simulink model "test_d_v_p_10_1"  (Simulink 7.0)
settings: Solver=ode45  StartTime=0.0  StopTime=30000  RelTol=1e-3
undefined symbols (not defined in the file): BEE2_usr, Down, Up
libraries: xbsIndex_r4 x479, xps_library x33, xbsReplacements_r4 x19, casper_library x15
(part 2 of 4)

== system test_d_v_p_10_1/pulse_ext1 ==
  in : Inport  OutDataType=sfix(16)  OutScaling=2^0
  Constant : xbsIndex_r4/Constant  arith_type=Boolean  const=1  n_bits=1  bin_pt=0  explicit_period=off  period=1  equ=P=C  opselect=C  inp2=PCIN>>17  opr=+  inp1=P  carry=CIN  dbl_ovrd=off  block_type=constant
  Constant17 : xbsIndex_r4/Constant  arith_type=Unsigned  const=pulse_len  n_bits=bits  bin_pt=0  explicit_period=on  period=1  equ=P=C  opselect=C  inp2=PCIN>>17  opr=+  inp1=P  carry=CIN  dbl_ovrd=off  block_type=constant
  Relational1 : xbsIndex_r4/Relational  mode=a<b  en=off  latency=0  dbl_ovrd=off  block_type=relational
      settings: xl_area=[0, 0, 0, 0, 0, 0, 0]  block_version=10.1.3
  Terminator : Terminator
  freeze_cntr : Subsystem  mask{CounterBits=bits}
      mask prompts: CounterBits "Counter Length (2^?)"
  posedge : Subsystem  Tag=Rising Edge Detector
  out : Outport  OutDataType=sfix(16)  OutScaling=2^0
  wires:
  Constant/1 -> freeze_cntr/1(en)
  freeze_cntr/2(we) -> Terminator/1
  freeze_cntr/1(addr) -> Relational1/1
  posedge/1(Out) -> freeze_cntr/2(rst)
  Constant17/1 -> Relational1/2
  Relational1/1 -> out/1
  in/1 -> posedge/1(In)

== system test_d_v_p_10_1/pulse_ext2 ==
  in : Inport  OutDataType=sfix(16)  OutScaling=2^0
  Constant : xbsIndex_r4/Constant  arith_type=Boolean  const=1  n_bits=1  bin_pt=0  explicit_period=off  period=1  equ=P=C  opselect=C  inp2=PCIN>>17  opr=+  inp1=P  carry=CIN  dbl_ovrd=off  block_type=constant
  Constant17 : xbsIndex_r4/Constant  arith_type=Unsigned  const=pulse_len  n_bits=bits  bin_pt=0  explicit_period=on  period=1  equ=P=C  opselect=C  inp2=PCIN>>17  opr=+  inp1=P  carry=CIN  dbl_ovrd=off  block_type=constant
  Relational1 : xbsIndex_r4/Relational  mode=a<b  en=off  latency=0  dbl_ovrd=off  block_type=relational
      settings: xl_area=[0, 0, 0, 0, 0, 0, 0]  block_version=10.1.3
  Terminator : Terminator
  freeze_cntr : Subsystem  mask{CounterBits=bits}
      mask prompts: CounterBits "Counter Length (2^?)"
  posedge : Subsystem  Tag=Rising Edge Detector
  out : Outport  OutDataType=sfix(16)  OutScaling=2^0
  wires:
  Constant/1 -> freeze_cntr/1(en)
  freeze_cntr/2(we) -> Terminator/1
  freeze_cntr/1(addr) -> Relational1/1
  posedge/1(Out) -> freeze_cntr/2(rst)
  Constant17/1 -> Relational1/2
  Relational1/1 -> out/1
  in/1 -> posedge/1(In)

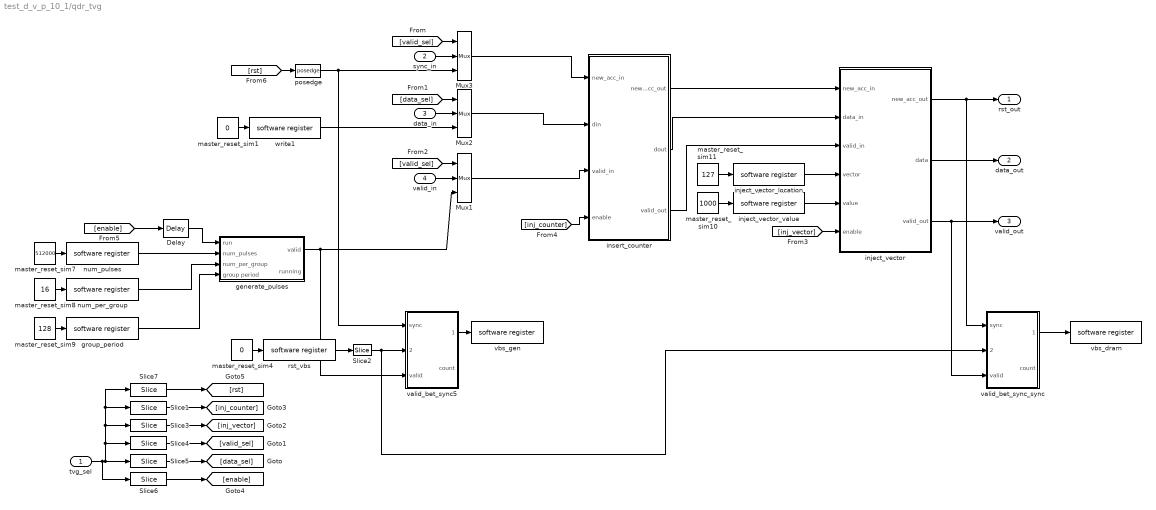
== system test_d_v_p_10_1/qdr_tvg ==
  tvg_sel : Inport  OutDataType=sfix(16)  OutScaling=2^0
  sync_in : Inport  Port=2  OutDataType=sfix(16)  OutScaling=2^0
  data_in : Inport  Port=3  OutDataType=sfix(16)  OutScaling=2^0
  valid_in : Inport  Port=4  OutDataType=sfix(16)  OutScaling=2^0
  Delay : xbsIndex_r4/Delay  en=off  latency=1  dbl_ovrd=off  reg_retiming=on  block_type=delay
      settings: xl_area=[0, 0, 0, 0, 0, 0, 0]
  Mux1 : xbsIndex_r4/Mux  inputs=2  en=off  latency=0  precision=Full  arith_type="Signed  (2's comp)"  n_bits=8  bin_pt=2  quantization=Truncate  overflow=Wrap  dbl_ovrd=off  block_type=mux
      settings: xl_area=[0, 0, 0, 0, 0, 0, 0]
  Mux2 : xbsIndex_r4/Mux  inputs=2  en=off  latency=0  precision=Full  arith_type="Signed  (2's comp)"  n_bits=8  bin_pt=2  quantization=Truncate  overflow=Wrap  dbl_ovrd=off  block_type=mux
      settings: xl_area=[0, 0, 0, 0, 0, 0, 0]
  Mux3 : xbsIndex_r4/Mux  inputs=2  en=off  latency=0  precision=Full  arith_type="Signed  (2's comp)"  n_bits=8  bin_pt=2  quantization=Truncate  overflow=Wrap  dbl_ovrd=off  block_type=mux
      settings: xl_area=[0, 0, 0, 0, 0, 0, 0]
  Slice1 : xbsIndex_r4/Slice  nbits=1  boolean_output=on  mode=Lower Bit Location + Width  bit1=0  base1=MSB of Input  bit0=4  base0=LSB of Input  dbl_ovrd=off  block_type=slice
      settings: infoedit="Extracts a given range of bits from each input sample and presents it at the output.  The output type is ordinarily unsigned with binary point at zero, but can be Boolean when the slice is one bit wide.<P><P>Hardware notes: In hardware this block costs nothing."  block_version=10.1.3
  Slice2 : xbsIndex_r4/Slice  nbits=1  boolean_output=on  mode=Lower Bit Location + Width  bit1=0  base1=MSB of Input  bit0=0  base0=LSB of Input  dbl_ovrd=off  block_type=slice
      settings: infoedit="Extracts a given range of bits from each input sample and presents it at the output.  The output type is ordinarily unsigned with binary point at zero, but can be Boolean when the slice is one bit wide.<P><P>Hardware notes: In hardware this block costs nothing."  block_version=10.1.3
  Slice3 : xbsIndex_r4/Slice  nbits=1  boolean_output=on  mode=Lower Bit Location + Width  bit1=0  base1=MSB of Input  bit0=3  base0=LSB of Input  dbl_ovrd=off  block_type=slice
      settings: infoedit="Extracts a given range of bits from each input sample and presents it at the output.  The output type is ordinarily unsigned with binary point at zero, but can be Boolean when the slice is one bit wide.<P><P>Hardware notes: In hardware this block costs nothing."  block_version=10.1.3
  Slice4 : xbsIndex_r4/Slice  nbits=1  boolean_output=on  mode=Lower Bit Location + Width  bit1=0  base1=MSB of Input  bit0=2  base0=LSB of Input  dbl_ovrd=off  block_type=slice
      settings: infoedit="Extracts a given range of bits from each input sample and presents it at the output.  The output type is ordinarily unsigned with binary point at zero, but can be Boolean when the slice is one bit wide.<P><P>Hardware notes: In hardware this block costs nothing."  block_version=10.1.3
  Slice5 : xbsIndex_r4/Slice  nbits=1  boolean_output=on  mode=Lower Bit Location + Width  bit1=0  base1=MSB of Input  bit0=1  base0=LSB of Input  dbl_ovrd=off  block_type=slice
      settings: infoedit="Extracts a given range of bits from each input sample and presents it at the output.  The output type is ordinarily unsigned with binary point at zero, but can be Boolean when the slice is one bit wide.<P><P>Hardware notes: In hardware this block costs nothing."  block_version=10.1.3
  Slice6 : xbsIndex_r4/Slice  nbits=1  boolean_output=on  mode=Lower Bit Location + Width  bit1=0  base1=MSB of Input  bit0=0  base0=LSB of Input  dbl_ovrd=off  block_type=slice
      settings: infoedit="Extracts a given range of bits from each input sample and presents it at the output.  The output type is ordinarily unsigned with binary point at zero, but can be Boolean when the slice is one bit wide.<P><P>Hardware notes: In hardware this block costs nothing."  block_version=10.1.3
  Slice7 : xbsIndex_r4/Slice  nbits=1  boolean_output=on  mode=Lower Bit Location + Width  bit1=0  base1=MSB of Input  bit0=5  base0=LSB of Input  dbl_ovrd=off  block_type=slice
      settings: infoedit="Extracts a given range of bits from each input sample and presents it at the output.  The output type is ordinarily unsigned with binary point at zero, but can be Boolean when the slice is one bit wide.<P><P>Hardware notes: In hardware this block costs nothing."  block_version=10.1.3
  generate_pulses : Subsystem
  group_period : xps_library/software register  Tag=xps:sw_reg  SystemSampleTime=-1  io_dir=From Processor  arith_type=Unsigned  bitwidth=32  bin_pt=0  sample_period=1  gw_name=test_d_v_p_10_1_qdr_tvg_group_period_user_data_out
      link override qdr_vacc_dram_tvg1_group_period_user_data_out: arith_type=Unsigned  n_bits=32  bin_pt=0  period=1
      link override qdr_vacc_qdr_tvg_group_period_user_data_out: arith_type=Unsigned  n_bits=32  bin_pt=0  period=1
      link override test_qdr_vacc_qdr_tvg_group_period_user_data_out: arith_type=Unsigned  n_bits=32  bin_pt=0  period=1
  inject_vector : Subsystem  mask{num_vectors=len}
      mask prompts: num_vectors "number of vectors"
      mask init:
      | fmtstr = sprintf('Vector Length: %d', num_vectors);
      | set_param(gcb, 'AttributesFormatString', fmtstr);
      settings: AttributesFormatString=Vector Length: 150
  inject_vector_location : xps_library/software register  Tag=xps:sw_reg  SystemSampleTime=-1  io_dir=From Processor  arith_type=Unsigned  bitwidth=32  bin_pt=0  sample_period=1  gw_name=test_d_v_p_10_1_qdr_tvg_inject_vector_location_user_data_out
      link override qdr_vacc_dram_tvg1_inject_vector_location_user_data_out: arith_type=Unsigned  n_bits=32  bin_pt=0  period=1
      link override qdr_vacc_qdr_tvg_inject_vector_location_user_data_out: arith_type=Unsigned  n_bits=32  bin_pt=0  period=1
      link override test_qdr_vacc_qdr_tvg_inject_vector_location_user_data_out: arith_type=Unsigned  n_bits=32  bin_pt=0  period=1
  inject_vector_value : xps_library/software register  Tag=xps:sw_reg  SystemSampleTime=-1  io_dir=From Processor  arith_type="Signed  (2's comp)"  bitwidth=32  bin_pt=0  sample_period=1  gw_name=test_d_v_p_10_1_qdr_tvg_inject_vector_value_user_data_out
      link override qdr_vacc_dram_tvg1_inject_vector_value_user_data_out: arith_type=Unsigned  n_bits=32  bin_pt=0  period=1
      link override qdr_vacc_qdr_tvg_inject_vector_value_user_data_out: arith_type=Unsigned  n_bits=32  bin_pt=0  period=1
      link override test_qdr_vacc_qdr_tvg_inject_vector_value_user_data_out: arith_type="Signed  (2's comp)"  n_bits=32  bin_pt=0  period=1
  insert_counter : Subsystem  mask{vec_len=len}
      mask prompts: vec_len "Vector Length?"
      mask init:
      | fmtstr = sprintf('Vector Length: %d', vec_len);
      | set_param(gcb, 'AttributesFormatString', fmtstr);
      settings: AttributesFormatString=Vector Length: 150
  master_reset_sim1 : Constant  Value=0  OutDataType=sfix(16)  OutScaling=2^0
  master_reset_sim10 : Constant  Value=1000  OutDataType=sfix(16)  OutScaling=2^0
  master_reset_sim11 : Constant  Value=127  OutDataType=sfix(16)  OutScaling=2^0
  master_reset_sim4 : Constant  Value=0  OutDataType=sfix(16)  OutScaling=2^0
  master_reset_sim7 : Constant  Value=512000  OutDataType=sfix(16)  OutScaling=2^0
  master_reset_sim8 : Constant  Value=16  OutDataType=sfix(16)  OutScaling=2^0
  master_reset_sim9 : Constant  Value=128  OutDataType=sfix(16)  OutScaling=2^0
  num_per_group : xps_library/software register  Tag=xps:sw_reg  SystemSampleTime=-1  io_dir=From Processor  arith_type=Unsigned  bitwidth=32  bin_pt=0  sample_period=1  gw_name=test_d_v_p_10_1_qdr_tvg_num_per_group_user_data_out
      link override qdr_vacc_dram_tvg1_num_per_group_user_data_out: arith_type=Unsigned  n_bits=32  bin_pt=0  period=1
      link override qdr_vacc_qdr_tvg_num_per_group_user_data_out: arith_type=Unsigned  n_bits=32  bin_pt=0  period=1
      link override test_qdr_vacc_qdr_tvg_num_per_group_user_data_out: arith_type=Unsigned  n_bits=32  bin_pt=0  period=1
  num_pulses : xps_library/software register  Tag=xps:sw_reg  SystemSampleTime=-1  io_dir=From Processor  arith_type=Unsigned  bitwidth=32  bin_pt=0  sample_period=1  gw_name=test_d_v_p_10_1_qdr_tvg_num_pulses_user_data_out
      link override qdr_vacc_dram_tvg1_num_pulses_user_data_out: arith_type=Unsigned  n_bits=32  bin_pt=0  period=1
      link override qdr_vacc_qdr_tvg_num_pulses_user_data_out: arith_type=Unsigned  n_bits=32  bin_pt=0  period=1
      link override test_qdr_vacc_qdr_tvg_num_pulses_user_data_out: arith_type=Unsigned  n_bits=32  bin_pt=0  period=1
  posedge : casper_library/Misc/posedge  Tag=Rising Edge Detector  SystemSampleTime=-1
  rst_vbs : xps_library/software register  Tag=xps:sw_reg  SystemSampleTime=-1  io_dir=From Processor  arith_type=Unsigned  bitwidth=32  bin_pt=0  sample_period=1  gw_name=test_d_v_p_10_1_qdr_tvg_rst_vbs_user_data_out
      link override qdr_vacc_dram_tvg1_rst_vbs_user_data_out: arith_type=Unsigned  n_bits=32  bin_pt=0  period=1
      link override qdr_vacc_qdr_tvg_rst_vbs_user_data_out: arith_type=Unsigned  n_bits=32  bin_pt=0  period=1
      link override test_qdr_vacc_qdr_tvg_rst_vbs_user_data_out: arith_type=Unsigned  n_bits=32  bin_pt=0  period=1
  valid_bet_sync5 : Subsystem
  valid_bet_sync_sync : Subsystem
  vbs_dram : xps_library/software register  Tag=xps:sw_reg  SystemSampleTime=-1  io_dir=To Processor  arith_type=Unsigned  bitwidth=32  bin_pt=0  sample_period=1  gw_name=test_d_v_p_10_1_qdr_tvg_vbs_dram_user_data_in
      link override convert: arith_type=Unsigned  n_bits=32  bin_pt=0
  vbs_gen : xps_library/software register  Tag=xps:sw_reg  SystemSampleTime=-1  io_dir=To Processor  arith_type=Unsigned  bitwidth=32  bin_pt=0  sample_period=1  gw_name=test_d_v_p_10_1_qdr_tvg_vbs_gen_user_data_in
      link override convert: arith_type=Unsigned  n_bits=32  bin_pt=0
  write1 : xps_library/software register  Tag=xps:sw_reg  SystemSampleTime=-1  io_dir=From Processor  arith_type="Signed  (2's comp)"  bitwidth=32  bin_pt=0  sample_period=1  gw_name=test_d_v_p_10_1_qdr_tvg_write1_user_data_out
      link override qdr_vacc_dram_tvg1_write1_user_data_out: arith_type=Unsigned  n_bits=32  bin_pt=0  period=1
      link override qdr_vacc_qdr_tvg_write1_user_data_out: arith_type=Unsigned  n_bits=32  bin_pt=0  period=1
      link override test_qdr_vacc_qdr_tvg_write1_user_data_out: arith_type="Signed  (2's comp)"  n_bits=32  bin_pt=0  period=1
  rst_out : Outport  OutDataType=sfix(16)  OutScaling=2^0
  data_out : Outport  Port=2  OutDataType=sfix(16)  OutScaling=2^0
  valid_out : Outport  Port=3  OutDataType=sfix(16)  OutScaling=2^0
  wires:
  write1/1 -> Mux2/3
  master_reset_sim1/1 -> write1/1
  [rst] -> posedge/1
  num_pulses/1 -> generate_pulses/2(num_pulses)
  master_reset_sim7/1 -> num_pulses/1
  num_per_group/1 -> generate_pulses/3(num_per_group)
  master_reset_sim8/1 -> num_per_group/1
  group_period/1 -> generate_pulses/4(group period)
  master_reset_sim9/1 -> group_period/1
  Mux1/1 -> insert_counter/3(valid_in)
  valid_in/1 -> Mux1/2
  inject_vector/1(new_acc_out) -> rst_out/1, valid_bet_sync_sync/1(sync)
  inject_vector/2(data) -> data_out/1
  inject_vector/3(valid_out) -> valid_out/1, valid_bet_sync_sync/3(valid)
  insert_counter/1(new_acc_out) -> inject_vector/1(new_acc_in)
  Mux2/1 -> insert_counter/2(din)
  data_in/1 -> Mux2/2
  sync_in/1 -> Mux3/2
  Mux3/1 -> insert_counter/1(new_acc_in)
  Slice5/1 -> [data_sel]
  tvg_sel/1 -> Slice5/1, Slice3/1, Slice1/1, Slice7/1, Slice4/1, Slice6/1
  Slice4/1 -> [valid_sel]
  [valid_sel] -> Mux3/1
  [data_sel] -> Mux2/1
  [valid_sel] -> Mux1/1
  Slice3/1 -> [inj_vector]
  Slice1/1 -> [inj_counter]
  [enable] -> Delay/1
  insert_counter/2(dout) -> inject_vector/2(data_in)
  insert_counter/3(valid_out) -> inject_vector/3(valid_in)
  generate_pulses/1(valid) -> valid_bet_sync5/3(valid), Mux1/3
  posedge/1 -> valid_bet_sync5/1(sync), Mux3/3
  [inj_vector] -> inject_vector/6(enable)
  master_reset_sim11/1 -> inject_vector_location/1
  inject_vector_location/1 -> inject_vector/4(vector)
  master_reset_sim10/1 -> inject_vector_value/1
  inject_vector_value/1 -> inject_vector/5(value)
  [inj_counter] -> insert_counter/4(enable)
  Slice6/1 -> [enable]
  Slice7/1 -> [rst]
  valid_bet_sync5/1(max_count) -> vbs_gen/1
  master_reset_sim4/1 -> rst_vbs/1
  Slice2/1 -> valid_bet_sync5/2(rst_max), valid_bet_sync_sync/2(rst_max)
  rst_vbs/1 -> Slice2/1
  valid_bet_sync_sync/1(max_count) -> vbs_dram/1
  Delay/1 -> generate_pulses/1(run)

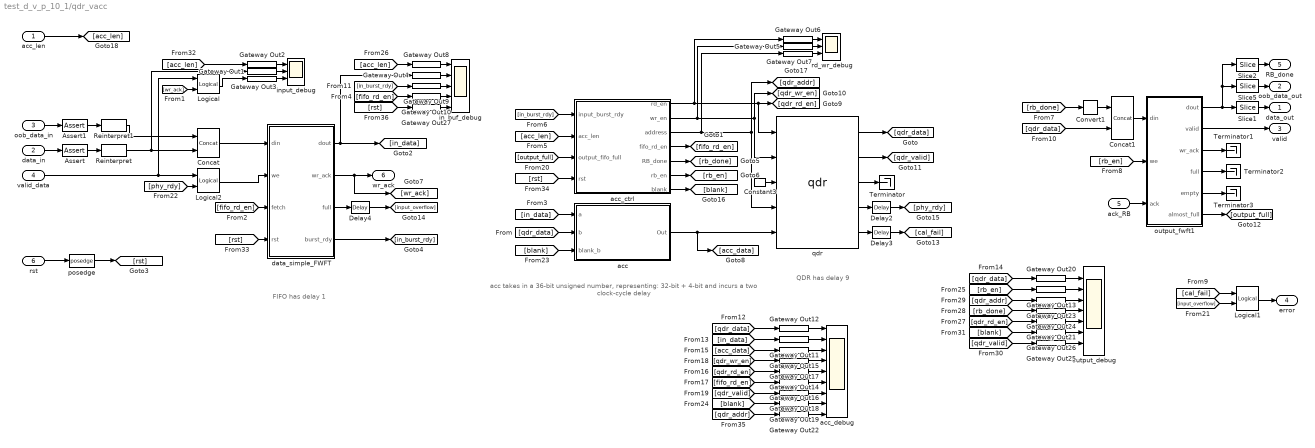
== system test_d_v_p_10_1/qdr_vacc ==
  note: QDR has delay 9
  note: FIFO has delay 1
  note: acc takes in a 36-bit unsigned
      | number, representing:
      | 32-bit + 4-bit and
      | incurs a two clock-cycle delay
  acc_len : Inport  OutDataType=sfix(16)  OutScaling=2^0
  data_in : Inport  Port=2  OutDataType=sfix(16)  OutScaling=2^0
  oob_data_in : Inport  Port=3  OutDataType=sfix(16)  OutScaling=2^0
  valid_data : Inport  Port=4  OutDataType=sfix(16)  OutScaling=2^0
  ack_RB : Inport  Port=5  OutDataType=sfix(16)  OutScaling=2^0
  rst : Inport  Port=6  OutDataType=sfix(16)  OutScaling=2^0
  Assert : xbsIndex_r4/Assert  assert_type=on  type_source=Explicitly  arith_type="Signed  (2's comp)"  n_bits=32  bin_pt=0  assert_rate=off  rate_source=Explicitly  period=1  output_port=on  block_type=assert
      settings: infoedit=Asserts a user-defined sample rate and/or type on a signal.<P><P>Hardware notes: In hardware this block costs nothing.  block_version=10.1.3
  Assert1 : xbsIndex_r4/Assert  assert_type=on  type_source=Explicitly  arith_type=Unsigned  n_bits=4  bin_pt=0  assert_rate=on  rate_source=Explicitly  period=1  output_port=on  block_type=assert
      settings: infoedit=Asserts a user-defined sample rate and/or type on a signal.<P><P>Hardware notes: In hardware this block costs nothing.  block_version=10.1.3
  Concat : xbsIndex_r4/Concat  num_inputs=2  dbl_ovrd=off  block_type=concat
      settings: block_version=9.2.01
  Concat1 : xbsIndex_r4/Concat  num_inputs=2  dbl_ovrd=off  block_type=concat
      settings: block_version=9.2.01
  Constant3 : xbsIndex_r4/Constant  arith_type=Unsigned  const=(2^4)-1  n_bits=4  bin_pt=0  explicit_period=on  period=1  equ=P=C  opselect=C  inp2=PCIN>>17  opr=+  inp1=P  carry=CIN  dbl_ovrd=off  block_type=constant
      settings: block_version=9.2.01
  Convert1 : xbsIndex_r4/Convert  arith_type=Unsigned  n_bits=1  bin_pt=0  quantization=Truncate  overflow=Wrap  latency=0  dbl_ovrd=off  pipeline=off  block_type=convert
      settings: xl_area=[0, 0, 0, 0, 0, 0, 0]  block_version=9.2.01
  Delay2 : xbsIndex_r4/Delay  en=off  latency=2  dbl_ovrd=off  reg_retiming=on  block_type=delay
  Delay3 : xbsIndex_r4/Delay  en=off  latency=2  dbl_ovrd=off  reg_retiming=on  block_type=delay
  Delay4 : xbsIndex_r4/Delay  en=off  latency=2  dbl_ovrd=off  reg_retiming=on  block_type=delay
  Gateway Out{1..27} (27 alike) : xbsIndex_r4/Gateway Out  hdl_port=on  timing_constraint=None  locs_specified=off  LOCs={}  block_type=gatewayout
      settings: infoedit="Gateway out block.  Converts Xilinx fixed point inputs into ouputs of type Simulink integer, double, or fixed point.<P><P>Hardware notes:  In hardware these blocks become top level output ports or are discarded, depending on how they are configured."  xl_area=[0, 0, 0, 0, 0, 0, 0]  block_version=10.1.3
  Logical : xbsIndex_r4/Logical  logical_function=AND  inputs=2  en=off  latency=0  precision=Full  arith_type=Unsigned  n_bits=16  bin_pt=0  align_bp=on  dbl_ovrd=off  block_type=logical
  Logical1 : xbsIndex_r4/Logical  logical_function=OR  inputs=2  en=off  latency=1  precision=Full  arith_type=Unsigned  n_bits=16  bin_pt=0  align_bp=on  dbl_ovrd=off  block_type=logical
  Logical2 : xbsIndex_r4/Logical  logical_function=AND  inputs=2  en=off  latency=0  precision=Full  arith_type=Unsigned  n_bits=16  bin_pt=0  align_bp=on  dbl_ovrd=off  block_type=logical
  Reinterpret : xbsIndex_r4/Reinterpret  force_arith_type=on  arith_type=Unsigned  force_bin_pt=on  bin_pt=0  block_type=reinterpret
      settings: infoedit="Changes signal type without altering the binary representation.   You can changed the signal between signed and unsigned, and relocate the binary point.<P><P>Hardware notes: In hardware this block costs nothing.<P><P>Example:  Suppose the input is 6 bits wide, signed, with 2 fractional bits, and the output is forced to unsigned with 0 fractional bits.  Then an input of -2.0 (1110.00 in binary 2's complement) becomes an output of 56 (111000 in binary)."  block_version=9.2.01
  Reinterpret1 : xbsIndex_r4/Reinterpret  force_arith_type=on  arith_type=Unsigned  force_bin_pt=on  bin_pt=0  block_type=reinterpret
      settings: infoedit="Changes signal type without altering the binary representation.   You can changed the signal between signed and unsigned, and relocate the binary point.<P><P>Hardware notes: In hardware this block costs nothing.<P><P>Example:  Suppose the input is 6 bits wide, signed, with 2 fractional bits, and the output is forced to unsigned with 0 fractional bits.  Then an input of -2.0 (1110.00 in binary 2's complement) becomes an output of 56 (111000 in binary)."  block_version=9.2.01
  Slice1 : xbsIndex_r4/Slice  nbits=32  boolean_output=off  mode=Lower Bit Location + Width  bit1=96  base1=MSB of Input  bit0=0  base0=LSB of Input  dbl_ovrd=off  block_type=slice
      settings: infoedit="Extracts a given range of bits from each input sample and presents it at the output.  The output type is ordinarily unsigned with binary point at zero, but can be Boolean when the slice is one bit wide.<P><P>Hardware notes: In hardware this block costs nothing."  block_version=9.2.01
  Slice2 : xbsIndex_r4/Slice  nbits=1  boolean_output=on  mode=Lower Bit Location + Width  bit1=-1  base1=MSB of Input  bit0=36  base0=LSB of Input  dbl_ovrd=off  block_type=slice
      settings: infoedit="Extracts a given range of bits from each input sample and presents it at the output.  The output type is ordinarily unsigned with binary point at zero, but can be Boolean when the slice is one bit wide.<P><P>Hardware notes: In hardware this block costs nothing."  block_version=9.2.01
  Slice5 : xbsIndex_r4/Slice  nbits=4  boolean_output=off  mode=Lower Bit Location + Width  bit1=96  base1=MSB of Input  bit0=32  base0=LSB of Input  dbl_ovrd=off  block_type=slice
      settings: infoedit="Extracts a given range of bits from each input sample and presents it at the output.  The output type is ordinarily unsigned with binary point at zero, but can be Boolean when the slice is one bit wide.<P><P>Hardware notes: In hardware this block costs nothing."  block_version=9.2.01
  Terminator{,1..3} (4 alike) : Terminator
  acc : Subsystem
  acc_ctrl : Subsystem
  acc_debug : Scope  NumInputPorts=9
      settings: TimeRange=57000  YMin=0~0~0~0~0~0~0~0~0  YMax=3000~1000~3000~1~1~1~1~1~150  SaveName=ScopeData4
  data_simple_FWFT : Subsystem  mask{burst_bits=burst_bits}
      mask prompts: burst_bits "Burst Length (2^?)"
      mask help: A rollback fifo behaves as a normal fifo, except that data which are written in have to be "committed" before they become available for readout. Moreover, any data which are written in and have not been committed can be "discarded", and will never be made available for readout.
      mask init:
      | fmtstr = sprintf('Depth: %d', 2^(burst_bits+2));
      | set_param(gcb, 'AttributesFormatString', fmtstr);
      settings: AttributesFormatString=Depth: 64
  in_buf_debug : Scope  NumInputPorts=5
      settings: YMin=12000~0~-5~-5~-5  YMax=13300~1~5~5~5  SaveName=ScopeData2
  input_debug : Scope  NumInputPorts=3
      settings: YMin=12000~0~-5  YMax=13300~1~5
  output_debug : Scope  NumInputPorts=7
      settings: YMin=0~0~0~0~0~0~0  YMax=600~1~225~1~1~1~1  SaveName=ScopeData3
  output_fwft1 : Subsystem  mask{depth_bits=10, burst_bits=burst_bits}
      mask prompts: depth_bits "Fifo Depth (2^?):"; burst_bits "Almost full warning (2^?)"
      mask help: A rollback fifo behaves as a normal fifo, except that data which are written in have to be "committed" before they become available for readout. Moreover, any data which are written in and have not been committed can be "discarded", and will never be made available for readout.
      mask init:
      | fmtstr = sprintf('Depth: %d', 2^depth_bits);
      | set_param(gcb, 'AttributesFormatString', fmtstr);
      settings: AttributesFormatString=Depth: 1024
  posedge : casper_library/Misc/posedge  Tag=Rising Edge Detector  SystemSampleTime=-1
  qdr : xps_library/qdr  Tag=xps:qdr  SystemSampleTime=-1  which_qdr=qdr0  qdr_awidth=12
  rd_wr_debug : Scope  NumInputPorts=3
      settings: YMin=12000~0~-5  YMax=13300~1~5
  data_out : Outport  OutDataType=sfix(16)  OutScaling=2^0
  oob_data_out : Outport  Port=2  OutDataType=sfix(16)  OutScaling=2^0
  valid : Outport  Port=3  OutDataType=sfix(16)  OutScaling=2^0
  error : Outport  Port=4  OutDataType=sfix(16)  OutScaling=2^0
  RB_done : Outport  Port=5  OutDataType=sfix(16)  OutScaling=2^0
  wr_ack : Outport  Port=6  OutDataType=sfix(16)  OutScaling=2^0
  wires:
  data_in/1 -> Assert/1
  valid_data/1 -> Logical/1, Logical2/1
  Concat/1 -> data_simple_FWFT/1(din)
  data_simple_FWFT/2(wr_ack) -> wr_ack/1, [wr_ack]
  acc_ctrl/1(rd_en) -> Gateway Out6/1, [qdr_rd_en], qdr/1
  acc_ctrl/2(wr_en) -> Gateway Out5/1, [qdr_wr_en], qdr/2
  acc_ctrl/3(address) -> Gateway Out7/1, [qdr_addr], qdr/4
  qdr/1 -> [qdr_data]
  Constant3/1 -> qdr/3
  acc_ctrl/4(fifo_rd_en) -> [fifo_rd_en]
  [fifo_rd_en] -> data_simple_FWFT/3(fetch)
  data_simple_FWFT/1(dout) -> Gateway Out4/1, [in_data]
  [in_burst_rdy] -> acc_ctrl/1(input_burst_rdy)
  data_simple_FWFT/4(burst_rdy) -> [in_burst_rdy]
  output_fwft1/2(valid) -> valid/1
  ack_RB/1 -> output_fwft1/3(ack)
  [rb_en] -> output_fwft1/2(we)
  [qdr_data] -> Concat1/2
  Concat1/1 -> output_fwft1/1(din)
  [rb_done] -> Convert1/1
  Convert1/1 -> Concat1/1
  output_fwft1/1(dout) -> Slice1/1, Slice2/1, Slice5/1
  Slice2/1 -> RB_done/1
  Slice1/1 -> data_out/1
  Gateway Out6/1 -> rd_wr_debug/1
  Gateway Out5/1 -> rd_wr_debug/2
  Gateway Out7/1 -> rd_wr_debug/3
  acc/1(Out) -> [acc_data], qdr/5
  Gateway Out2/1 -> input_debug/1
  Gateway Out1/1 -> input_debug/2
  Gateway Out3/1 -> input_debug/3
  Logical/1 -> Gateway Out3/1
  [wr_ack] -> Logical/2
  Gateway Out8/1 -> in_buf_debug/1
  Gateway Out4/1 -> in_buf_debug/2
  Gateway Out9/1 -> in_buf_debug/3
  Gateway Out10/1 -> in_buf_debug/4
  [fifo_rd_en] -> Gateway Out10/1
  [in_burst_rdy] -> Gateway Out9/1
  Slice5/1 -> oob_data_out/1
  [qdr_data] -> Gateway Out12/1
  [in_data] -> Gateway Out11/1
  [acc_data] -> Gateway Out15/1
  [qdr_rd_en] -> Gateway Out14/1
  [fifo_rd_en] -> Gateway Out16/1
  [qdr_wr_en] -> Gateway Out17/1
  qdr/2 -> [qdr_valid]
  [qdr_valid] -> Gateway Out18/1
  [output_full] -> acc_ctrl/3(output_fifo_full)
  output_fwft1/6(almost_full) -> [output_full]
  acc_ctrl/6(rb_en) -> [rb_en]
  acc_ctrl/5(RB_done) -> [rb_done]
  Logical1/1 -> error/1
  qdr/5 -> Delay3/1
  data_simple_FWFT/3(full) -> Delay4/1
  qdr/4 -> Delay2/1
  Delay2/1 -> [phy_rdy]
  Delay3/1 -> [cal_fail]
  [cal_fail] -> Logical1/1
  [input_overflow] -> Logical1/2
  Delay4/1 -> [input_overflow]
  Logical2/1 -> data_simple_FWFT/2(we)
  [phy_rdy] -> Logical2/2
  qdr/3 -> Terminator/1
  output_fwft1/3(wr_ack) -> Terminator1/1
  output_fwft1/4(full) -> Terminator2/1
  output_fwft1/5(empty) -> Terminator3/1
  [qdr_data] -> acc/2(b)
  acc_ctrl/7(blank) -> [blank]
  [blank] -> acc/3(blank_b)
  [blank] -> Gateway Out19/1
  Gateway Out12/1 -> acc_debug/1
  Gateway Out11/1 -> acc_debug/2
  Gateway Out15/1 -> acc_debug/3
  Gateway Out17/1 -> acc_debug/4
  Gateway Out14/1 -> acc_debug/5
  Gateway Out16/1 -> acc_debug/6
  Gateway Out18/1 -> acc_debug/7
  Gateway Out19/1 -> acc_debug/8
  [qdr_data] -> Gateway Out20/1
  [qdr_rd_en] -> Gateway Out21/1
  [qdr_valid] -> Gateway Out25/1
  [blank] -> Gateway Out26/1
  Gateway Out20/1 -> output_debug/1
  Gateway Out13/1 -> output_debug/2
  Gateway Out24/1 -> output_debug/4
  Gateway Out21/1 -> output_debug/5
  Gateway Out25/1 -> output_debug/7
  [rb_en] -> Gateway Out13/1
  [rb_done] -> Gateway Out24/1
  Gateway Out26/1 -> output_debug/6
  [qdr_addr] -> Gateway Out23/1
  Gateway Out23/1 -> output_debug/3
  acc_len/1 -> [acc_len]
  oob_data_in/1 -> Assert1/1
  [acc_len] -> acc_ctrl/2(acc_len)
  [acc_len] -> Gateway Out8/1
  [acc_len] -> Gateway Out2/1
  [rst] -> data_simple_FWFT/4(rst)
  [rst] -> acc_ctrl/4(rst)
  [qdr_addr] -> Gateway Out22/1
  Gateway Out22/1 -> acc_debug/9
  Gateway Out27/1 -> in_buf_debug/5
  [rst] -> Gateway Out27/1
  rst/1 -> posedge/1
  posedge/1 -> [rst]
  [in_data] -> acc/1(a)
  Assert/1 -> Reinterpret/1
  Assert1/1 -> Reinterpret1/1
  Reinterpret/1 -> Gateway Out1/1, Concat/2
  Reinterpret1/1 -> Concat/1

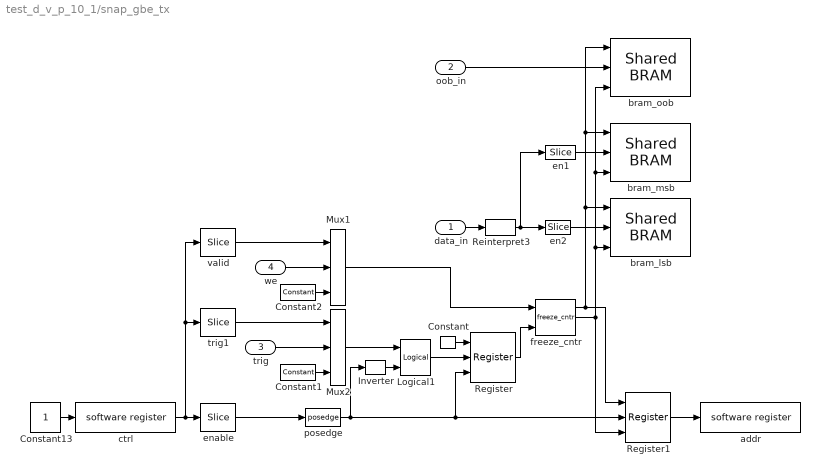
== system test_d_v_p_10_1/snap_gbe_tx ==
  data_in : Inport  OutDataType=sfix(16)  OutScaling=2^0
  oob_in : Inport  Port=2  OutDataType=sfix(16)  OutScaling=2^0
  trig : Inport  Port=3  OutDataType=sfix(16)  OutScaling=2^0
  we : Inport  Port=4  OutDataType=sfix(16)  OutScaling=2^0
  Constant : xbsIndex_r4/Constant  arith_type=Boolean  const=1  n_bits=1  bin_pt=0  explicit_period=on  period=1  equ=P=C  opselect=C  inp2=PCIN>>17  opr=+  inp1=P  carry=CIN  dbl_ovrd=off  block_type=constant
  Constant1 : xbsIndex_r4/Constant  arith_type=Boolean  const=1  n_bits=1  bin_pt=0  explicit_period=on  period=1  equ=P=C  opselect=C  inp2=PCIN>>17  opr=+  inp1=P  carry=CIN  dbl_ovrd=off  block_type=constant
  Constant13 : Constant  OutDataType=sfix(16)  OutScaling=2^0
  Constant2 : xbsIndex_r4/Constant  arith_type=Boolean  const=1  n_bits=1  bin_pt=0  explicit_period=on  period=1  equ=P=C  opselect=C  inp2=PCIN>>17  opr=+  inp1=P  carry=CIN  dbl_ovrd=off  block_type=constant
  Inverter : xbsIndex_r4/Inverter  en=off  latency=0  dbl_ovrd=off  block_type=inv
      settings: xl_area=[0, 0, 0, 0, 0, 0, 0]
  Logical1 : xbsIndex_r4/Logical  logical_function=AND  inputs=2  en=off  latency=0  precision=Full  arith_type=Unsigned  n_bits=8  bin_pt=2  align_bp=on  dbl_ovrd=off  block_type=logical
      settings: xl_area=[0, 0, 0, 0, 0, 0, 0]
  Mux1 : xbsIndex_r4/Mux  inputs=2  en=off  latency=0  precision=Full  arith_type="Signed  (2's comp)"  n_bits=8  bin_pt=2  quantization=Truncate  overflow=Wrap  dbl_ovrd=off  block_type=mux
      settings: xl_area=[0, 0, 0, 0, 0, 0, 0]
  Mux2 : xbsIndex_r4/Mux  inputs=2  en=off  latency=0  precision=Full  arith_type="Signed  (2's comp)"  n_bits=8  bin_pt=2  quantization=Truncate  overflow=Wrap  dbl_ovrd=off  block_type=mux
      settings: xl_area=[0, 0, 0, 0, 0, 0, 0]
  Register : xbsIndex_r4/Register  init=0  rst=on  en=on  dbl_ovrd=off  block_type=register
      settings: xl_area=[0, 0, 0, 0, 0, 0, 0]
  Register1 : xbsIndex_r4/Register  init=0  rst=on  en=on  dbl_ovrd=off  block_type=register
      settings: xl_area=[0, 0, 0, 0, 0, 0, 0]
  Reinterpret3 : xbsIndex_r4/Reinterpret  force_arith_type=on  arith_type=Unsigned  force_bin_pt=on  bin_pt=0  block_type=reinterpret
      settings: infoedit="Changes signal type without altering the binary representation.   You can changed the signal between signed and unsigned, and relocate the binary point.<P><P>Hardware notes: In hardware this block costs nothing.<P><P>Example:  Suppose the input is 6 bits wide, signed, with 2 fractional bits, and the output is forced to unsigned with 0 fractional bits.  Then an input of -2.0 (1110.00 in binary 2's complement) becomes an output of 56 (111000 in binary)."  block_version=10.1.3
  addr : xps_library/software register  Tag=xps:sw_reg  SystemSampleTime=-1  io_dir=To Processor  arith_type=Unsigned  bitwidth=32  bin_pt=0  sample_period=1  gw_name=test_d_v_p_10_1_snap_gbe_tx_addr_user_data_in
  bram_lsb : xps_library/Shared BRAM  Tag=xps:bram  SystemSampleTime=-1  arith_type=Unsigned  addr_width=nsamples  data_width=32  data_bin_pt=0  init_vals=0  sample_rate=1
  bram_msb : xps_library/Shared BRAM  Tag=xps:bram  SystemSampleTime=-1  arith_type=Unsigned  addr_width=nsamples  data_width=32  data_bin_pt=0  init_vals=0  sample_rate=1
  bram_oob : xps_library/Shared BRAM  Tag=xps:bram  SystemSampleTime=-1  arith_type=Unsigned  addr_width=nsamples  data_width=32  data_bin_pt=0  init_vals=0  sample_rate=1
  ctrl : xps_library/software register  Tag=xps:sw_reg  SystemSampleTime=-1  io_dir=From Processor  arith_type=Unsigned  bitwidth=32  bin_pt=0  sample_period=1  gw_name=test_d_v_p_10_1_snap_gbe_tx_ctrl_user_data_out
  en1 : xbsIndex_r4/Slice  nbits=32  boolean_output=off  mode=Lower Bit Location + Width  bit1=0  base1=LSB of Input  bit0=32  base0=LSB of Input  dbl_ovrd=off  block_type=slice
      settings: infoedit="Extracts a given range of bits from each input sample and presents it at the output.  The output type is ordinarily unsigned with binary point at zero, but can be Boolean when the slice is one bit wide.<P><P>Hardware notes: In hardware this block costs nothing."  block_version=10.1.3
  en2 : xbsIndex_r4/Slice  nbits=32  boolean_output=off  mode=Lower Bit Location + Width  bit1=0  base1=LSB of Input  bit0=0  base0=LSB of Input  dbl_ovrd=off  block_type=slice
      settings: infoedit="Extracts a given range of bits from each input sample and presents it at the output.  The output type is ordinarily unsigned with binary point at zero, but can be Boolean when the slice is one bit wide.<P><P>Hardware notes: In hardware this block costs nothing."  block_version=10.1.3
  enable : xbsIndex_r4/Slice  nbits=1  boolean_output=on  mode=Lower Bit Location + Width  bit1=0  base1=LSB of Input  bit0=0  base0=LSB of Input  dbl_ovrd=off  block_type=slice
      settings: infoedit="Extracts a given range of bits from each input sample and presents it at the output.  The output type is ordinarily unsigned with binary point at zero, but can be Boolean when the slice is one bit wide.<P><P>Hardware notes: In hardware this block costs nothing."  block_version=10.1.3
  freeze_cntr : casper_library/Misc/freeze_cntr  SystemSampleTime=-1  CounterBits=nsamples
  posedge : casper_library/Misc/posedge  Tag=Rising Edge Detector  SystemSampleTime=-1
  trig1 : xbsIndex_r4/Slice  nbits=1  boolean_output=on  mode=Lower Bit Location + Width  bit1=0  base1=LSB of Input  bit0=1  base0=LSB of Input  dbl_ovrd=off  block_type=slice
      settings: infoedit="Extracts a given range of bits from each input sample and presents it at the output.  The output type is ordinarily unsigned with binary point at zero, but can be Boolean when the slice is one bit wide.<P><P>Hardware notes: In hardware this block costs nothing."  block_version=10.1.3
  valid : xbsIndex_r4/Slice  nbits=1  boolean_output=on  mode=Lower Bit Location + Width  bit1=0  base1=LSB of Input  bit0=2  base0=LSB of Input  dbl_ovrd=off  block_type=slice
      settings: infoedit="Extracts a given range of bits from each input sample and presents it at the output.  The output type is ordinarily unsigned with binary point at zero, but can be Boolean when the slice is one bit wide.<P><P>Hardware notes: In hardware this block costs nothing."  block_version=10.1.3
  wires:
  freeze_cntr/1 -> bram_lsb/1, bram_msb/1, bram_oob/1, Register1/1
  Register/1 -> freeze_cntr/2
  Mux2/1 -> Logical1/1
  Inverter/1 -> Logical1/2
  Logical1/1 -> Register/2
  valid/1 -> Mux1/1
  trig1/1 -> Mux2/1
  Register1/1 -> addr/1
  Constant2/1 -> Mux1/3
  we/1 -> Mux1/2
  Mux1/1 -> freeze_cntr/1
  Constant1/1 -> Mux2/3
  Constant/1 -> Register/1
  posedge/1 -> Inverter/1, Register1/2, Register/3
  ctrl/1 -> trig1/1, valid/1, enable/1
  Constant13/1 -> ctrl/1
  freeze_cntr/2 -> bram_lsb/3, bram_msb/3, bram_oob/3, Register1/3
  enable/1 -> posedge/1
  trig/1 -> Mux2/2
  Reinterpret3/1 -> en1/1, en2/1
  data_in/1 -> Reinterpret3/1
  en1/1 -> bram_msb/2
  en2/1 -> bram_lsb/2
  oob_in/1 -> bram_oob/2

== system test_d_v_p_10_1/xeng_label0 ==
  xeng_base : Inport  OutDataType=sfix(16)  OutScaling=2^0
  Concat : xbsIndex_r4/Concat  num_inputs=2  dbl_ovrd=off  block_type=concat
      settings: block_version=10.1.3
  Constant19 : xbsIndex_r4/Constant  arith_type=Unsigned  const=nx  n_bits=share_bits  bin_pt=0  explicit_period=on  period=1  equ=P=C  opselect=C  inp2=PCIN>>17  opr=+  inp1=P  carry=CIN  dbl_ovrd=off  block_type=constant
  Slice5 : xbsIndex_r4/Slice  nbits=16-share_bits  boolean_output=off  mode=Lower Bit Location + Width  bit1=0  base1=MSB of Input  bit0=share_bits  base0=LSB of Input  dbl_ovrd=off  block_type=slice
      settings: infoedit="Extracts a given range of bits from each input sample and presents it at the output.  The output type is ordinarily unsigned with binary point at zero, but can be Boolean when the slice is one bit wide.<P><P>Hardware notes: In hardware this block costs nothing."  block_version=10.1.3
  xeng : Outport  OutDataType=sfix(16)  OutScaling=2^0
  wires:
  Slice5/1 -> Concat/1
  Constant19/1 -> Concat/2
  xeng_base/1 -> Slice5/1
  Concat/1 -> xeng/1

== system test_d_v_p_10_1/Subsystem/data_sel1 ==
  In1 : Inport  OutDataType=sfix(16)  OutScaling=2^0
  Product : Product  OutDataType=sfix(16)  OutScaling=2^0  RndMeth=Zero
  err_clear_sim1 : Constant  Value=2^bit_pos  OutDataType=sfix(16)  OutScaling=2^0
  Out1 : Outport  OutDataType=sfix(16)  OutScaling=2^0
  wires:
  err_clear_sim1/1 -> Product/2
  In1/1 -> Product/1
  Product/1 -> Out1/1

== system test_d_v_p_10_1/Subsystem/inj_counter1 ==
  In1 : Inport  OutDataType=sfix(16)  OutScaling=2^0
  Product : Product  OutDataType=sfix(16)  OutScaling=2^0  RndMeth=Zero
  err_clear_sim1 : Constant  Value=2^bit_pos  OutDataType=sfix(16)  OutScaling=2^0
  Out1 : Outport  OutDataType=sfix(16)  OutScaling=2^0
  wires:
  err_clear_sim1/1 -> Product/2
  In1/1 -> Product/1
  Product/1 -> Out1/1

== system test_d_v_p_10_1/Subsystem/inj_vector1 ==
  In1 : Inport  OutDataType=sfix(16)  OutScaling=2^0
  Product : Product  OutDataType=sfix(16)  OutScaling=2^0  RndMeth=Zero
  err_clear_sim1 : Constant  Value=2^bit_pos  OutDataType=sfix(16)  OutScaling=2^0
  Out1 : Outport  OutDataType=sfix(16)  OutScaling=2^0
  wires:
  err_clear_sim1/1 -> Product/2
  In1/1 -> Product/1
  Product/1 -> Out1/1

== system test_d_v_p_10_1/Subsystem/new_acc2 ==
  In1 : Inport  OutDataType=sfix(16)  OutScaling=2^0
  Product : Product  OutDataType=sfix(16)  OutScaling=2^0  RndMeth=Zero
  err_clear_sim1 : Constant  Value=2^bit_pos  OutDataType=sfix(16)  OutScaling=2^0
  Out1 : Outport  OutDataType=sfix(16)  OutScaling=2^0
  wires:
  err_clear_sim1/1 -> Product/2
  In1/1 -> Product/1
  Product/1 -> Out1/1

== system test_d_v_p_10_1/Subsystem/run1 ==
  In1 : Inport  OutDataType=sfix(16)  OutScaling=2^0
  Product : Product  OutDataType=sfix(16)  OutScaling=2^0  RndMeth=Zero
  err_clear_sim1 : Constant  Value=2^bit_pos  OutDataType=sfix(16)  OutScaling=2^0
  Out1 : Outport  OutDataType=sfix(16)  OutScaling=2^0
  wires:
  err_clear_sim1/1 -> Product/2
  In1/1 -> Product/1
  Product/1 -> Out1/1

== system test_d_v_p_10_1/Subsystem/valid_sel1 ==
  In1 : Inport  OutDataType=sfix(16)  OutScaling=2^0
  Product : Product  OutDataType=sfix(16)  OutScaling=2^0  RndMeth=Zero
  err_clear_sim1 : Constant  Value=2^bit_pos  OutDataType=sfix(16)  OutScaling=2^0
  Out1 : Outport  OutDataType=sfix(16)  OutScaling=2^0
  wires:
  err_clear_sim1/1 -> Product/2
  In1/1 -> Product/1
  Product/1 -> Out1/1

== system test_d_v_p_10_1/pulse_ext/freeze_cntr ==
  en : Inport  OutDataType=sfix(16)  OutScaling=2^0
  rst : Inport  Port=2  OutDataType=sfix(16)  OutScaling=2^0
  Constant5 : xbsIndex_r4/Constant  arith_type=Unsigned  const=2^CounterBits - 1  n_bits=CounterBits  bin_pt=0  explicit_period=off  period=1  equ=P=C  opselect=C  inp2=PCIN>>17  opr=+  inp1=P  carry=CIN  dbl_ovrd=off  block_type=constant
  Counter3 : xbsIndex_r4/Counter  cnt_type=Free Running  cnt_to=1023  operation=Up  start_count=0  cnt_by_val=1  arith_type=Unsigned  n_bits=CounterBits  bin_pt=0  load_pin=off  rst=on  en=on  explicit_period=on  period=1  dbl_ovrd=off  use_behavioral_HDL=off  use_rpm=on  implementation=Fabric  block_type=counter
      settings: xl_area=[0, 0, 0, 0, 0, 0, 0]
  Inverter : xbsIndex_r4/Inverter  en=off  latency=0  dbl_ovrd=off  block_type=inv
      settings: xl_area=[0, 0, 0, 0, 0, 0, 0]
  Logical1 : xbsIndex_r4/Logical  logical_function=AND  inputs=2  en=off  latency=0  precision=Full  arith_type=Unsigned  n_bits=8  bin_pt=2  align_bp=on  dbl_ovrd=off  block_type=logical
      settings: xl_area=[0, 0, 0, 0, 0, 0, 0]
  Logical5 : xbsIndex_r4/Logical  logical_function=AND  inputs=2  en=off  latency=0  precision=Full  arith_type=Unsigned  n_bits=8  bin_pt=2  align_bp=on  dbl_ovrd=off  block_type=logical
      settings: xl_area=[0, 0, 0, 0, 0, 0, 0]
  Relational5 : xbsIndex_r4/Relational  mode=a!=b  en=off  latency=0  dbl_ovrd=off  block_type=relational
      settings: xl_area=[0, 0, 0, 0, 0, 0, 0]  block_version=10.1.3
  addr : Outport  OutDataType=sfix(16)  OutScaling=2^0
  we : Outport  Port=2  OutDataType=sfix(16)  OutScaling=2^0
  wires:
  rst/1 -> Counter3/1, Inverter/1
  Logical5/1 -> Counter3/2, Logical1/2
  en/1 -> Logical5/1
  Relational5/1 -> Logical5/2
  Constant5/1 -> Relational5/2
  Counter3/1 -> Relational5/1, addr/1
  Inverter/1 -> Logical1/1
  Logical1/1 -> we/1

== system test_d_v_p_10_1/pulse_ext/posedge ==
  In : Inport  OutDataType=sfix(16)  OutScaling=2^0
  Delay : xbsIndex_r4/Delay  en=off  latency=1  dbl_ovrd=off  reg_retiming=off  block_type=delay
      settings: xl_area=[0, 0, 0, 0, 0, 0, 0]
  Inverter : xbsIndex_r4/Inverter  en=off  latency=0  dbl_ovrd=off  block_type=inv
      settings: xl_area=[0, 0, 0, 0, 0, 0, 0]
  Logical : xbsIndex_r4/Logical  logical_function=AND  inputs=2  en=off  latency=0  precision=Full  arith_type=Unsigned  n_bits=8  bin_pt=2  align_bp=on  dbl_ovrd=off  block_type=logical
      settings: xl_area=[0, 0, 0, 0, 0, 0, 0]
  Out : Outport  OutDataType=sfix(16)  OutScaling=2^0
  wires:
  Delay/1 -> Inverter/1
  Inverter/1 -> Logical/1
  In/1 -> Delay/1, Logical/2
  Logical/1 -> Out/1

== system test_d_v_p_10_1/pulse_ext1/freeze_cntr ==
  en : Inport  OutDataType=sfix(16)  OutScaling=2^0
  rst : Inport  Port=2  OutDataType=sfix(16)  OutScaling=2^0
  Constant5 : xbsIndex_r4/Constant  arith_type=Unsigned  const=2^CounterBits - 1  n_bits=CounterBits  bin_pt=0  explicit_period=off  period=1  equ=P=C  opselect=C  inp2=PCIN>>17  opr=+  inp1=P  carry=CIN  dbl_ovrd=off  block_type=constant
  Counter3 : xbsIndex_r4/Counter  cnt_type=Free Running  cnt_to=1023  operation=Up  start_count=0  cnt_by_val=1  arith_type=Unsigned  n_bits=CounterBits  bin_pt=0  load_pin=off  rst=on  en=on  explicit_period=on  period=1  dbl_ovrd=off  use_behavioral_HDL=off  use_rpm=on  implementation=Fabric  block_type=counter
      settings: xl_area=[0, 0, 0, 0, 0, 0, 0]
  Inverter : xbsIndex_r4/Inverter  en=off  latency=0  dbl_ovrd=off  block_type=inv
      settings: xl_area=[0, 0, 0, 0, 0, 0, 0]
  Logical1 : xbsIndex_r4/Logical  logical_function=AND  inputs=2  en=off  latency=0  precision=Full  arith_type=Unsigned  n_bits=8  bin_pt=2  align_bp=on  dbl_ovrd=off  block_type=logical
      settings: xl_area=[0, 0, 0, 0, 0, 0, 0]
  Logical5 : xbsIndex_r4/Logical  logical_function=AND  inputs=2  en=off  latency=0  precision=Full  arith_type=Unsigned  n_bits=8  bin_pt=2  align_bp=on  dbl_ovrd=off  block_type=logical
      settings: xl_area=[0, 0, 0, 0, 0, 0, 0]
  Relational5 : xbsIndex_r4/Relational  mode=a!=b  en=off  latency=0  dbl_ovrd=off  block_type=relational
      settings: xl_area=[0, 0, 0, 0, 0, 0, 0]  block_version=10.1.3
  addr : Outport  OutDataType=sfix(16)  OutScaling=2^0
  we : Outport  Port=2  OutDataType=sfix(16)  OutScaling=2^0
  wires:
  rst/1 -> Counter3/1, Inverter/1
  Logical5/1 -> Counter3/2, Logical1/2
  en/1 -> Logical5/1
  Relational5/1 -> Logical5/2
  Constant5/1 -> Relational5/2
  Counter3/1 -> Relational5/1, addr/1
  Inverter/1 -> Logical1/1
  Logical1/1 -> we/1

== system test_d_v_p_10_1/pulse_ext1/posedge ==
  In : Inport  OutDataType=sfix(16)  OutScaling=2^0
  Delay : xbsIndex_r4/Delay  en=off  latency=1  dbl_ovrd=off  reg_retiming=off  block_type=delay
      settings: xl_area=[0, 0, 0, 0, 0, 0, 0]
  Inverter : xbsIndex_r4/Inverter  en=off  latency=0  dbl_ovrd=off  block_type=inv
      settings: xl_area=[0, 0, 0, 0, 0, 0, 0]
  Logical : xbsIndex_r4/Logical  logical_function=AND  inputs=2  en=off  latency=0  precision=Full  arith_type=Unsigned  n_bits=8  bin_pt=2  align_bp=on  dbl_ovrd=off  block_type=logical
      settings: xl_area=[0, 0, 0, 0, 0, 0, 0]
  Out : Outport  OutDataType=sfix(16)  OutScaling=2^0
  wires:
  Delay/1 -> Inverter/1
  Inverter/1 -> Logical/1
  In/1 -> Delay/1, Logical/2
  Logical/1 -> Out/1

== system test_d_v_p_10_1/pulse_ext2/freeze_cntr ==
  en : Inport  OutDataType=sfix(16)  OutScaling=2^0
  rst : Inport  Port=2  OutDataType=sfix(16)  OutScaling=2^0
  Constant5 : xbsIndex_r4/Constant  arith_type=Unsigned  const=2^CounterBits - 1  n_bits=CounterBits  bin_pt=0  explicit_period=off  period=1  equ=P=C  opselect=C  inp2=PCIN>>17  opr=+  inp1=P  carry=CIN  dbl_ovrd=off  block_type=constant
  Counter3 : xbsIndex_r4/Counter  cnt_type=Free Running  cnt_to=1023  operation=Up  start_count=0  cnt_by_val=1  arith_type=Unsigned  n_bits=CounterBits  bin_pt=0  load_pin=off  rst=on  en=on  explicit_period=on  period=1  dbl_ovrd=off  use_behavioral_HDL=off  use_rpm=on  implementation=Fabric  block_type=counter
      settings: xl_area=[0, 0, 0, 0, 0, 0, 0]
  Inverter : xbsIndex_r4/Inverter  en=off  latency=0  dbl_ovrd=off  block_type=inv
      settings: xl_area=[0, 0, 0, 0, 0, 0, 0]
  Logical1 : xbsIndex_r4/Logical  logical_function=AND  inputs=2  en=off  latency=0  precision=Full  arith_type=Unsigned  n_bits=8  bin_pt=2  align_bp=on  dbl_ovrd=off  block_type=logical
      settings: xl_area=[0, 0, 0, 0, 0, 0, 0]
  Logical5 : xbsIndex_r4/Logical  logical_function=AND  inputs=2  en=off  latency=0  precision=Full  arith_type=Unsigned  n_bits=8  bin_pt=2  align_bp=on  dbl_ovrd=off  block_type=logical
      settings: xl_area=[0, 0, 0, 0, 0, 0, 0]
  Relational5 : xbsIndex_r4/Relational  mode=a!=b  en=off  latency=0  dbl_ovrd=off  block_type=relational
      settings: xl_area=[0, 0, 0, 0, 0, 0, 0]  block_version=10.1.3
  addr : Outport  OutDataType=sfix(16)  OutScaling=2^0
  we : Outport  Port=2  OutDataType=sfix(16)  OutScaling=2^0
  wires:
  rst/1 -> Counter3/1, Inverter/1
  Logical5/1 -> Counter3/2, Logical1/2
  en/1 -> Logical5/1
  Relational5/1 -> Logical5/2
  Constant5/1 -> Relational5/2
  Counter3/1 -> Relational5/1, addr/1
  Inverter/1 -> Logical1/1
  Logical1/1 -> we/1

== system test_d_v_p_10_1/pulse_ext2/posedge ==
  In : Inport  OutDataType=sfix(16)  OutScaling=2^0
  Delay : xbsIndex_r4/Delay  en=off  latency=1  dbl_ovrd=off  reg_retiming=off  block_type=delay
      settings: xl_area=[0, 0, 0, 0, 0, 0, 0]
  Inverter : xbsIndex_r4/Inverter  en=off  latency=0  dbl_ovrd=off  block_type=inv
      settings: xl_area=[0, 0, 0, 0, 0, 0, 0]
  Logical : xbsIndex_r4/Logical  logical_function=AND  inputs=2  en=off  latency=0  precision=Full  arith_type=Unsigned  n_bits=8  bin_pt=2  align_bp=on  dbl_ovrd=off  block_type=logical
      settings: xl_area=[0, 0, 0, 0, 0, 0, 0]
  Out : Outport  OutDataType=sfix(16)  OutScaling=2^0
  wires:
  Delay/1 -> Inverter/1
  Inverter/1 -> Logical/1
  In/1 -> Delay/1, Logical/2
  Logical/1 -> Out/1
